simulink model "SIRModell"  (R2024b)
settings: Solver=VariableStepAuto  StartTime=0.0  StopTime=365  RelTol=1e-3
settings Model: Creator=castl  LastModifiedBy=castl

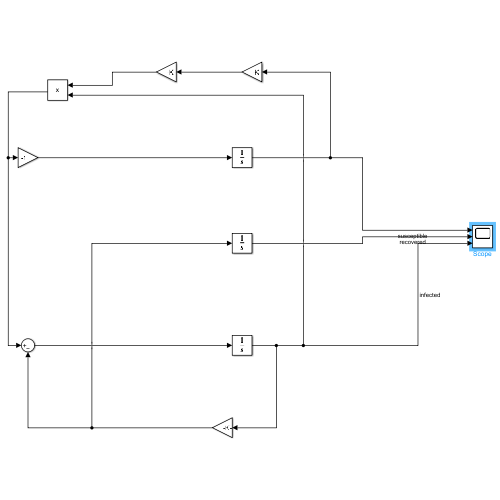
[thumbnail: Simulink's stored preview of the top-level diagram]
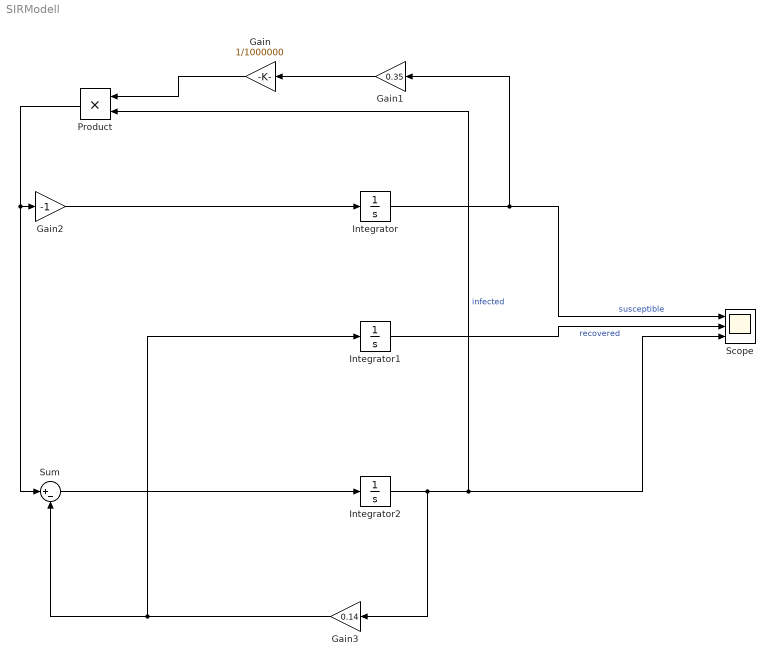
== system SIRModell ==
  Gain : Gain  Gain=1/1000000
  Gain1 : Gain  Gain=0.35
  Gain2 : Gain  Gain=-1
  Gain3 : Gain  Gain=0.14
  Integrator : Integrator  InitialCondition=999833
  Integrator1 : Integrator  InitialCondition=1
  Integrator2 : Integrator  InitialCondition=166
  Product : Product
  Scope : Scope  NumInputPorts=3
  Sum : Sum  Inputs=|+-
  wires:
  Gain2/1 -> Integrator/1
  Sum/1 -> Integrator2/1
  Gain3/1 -> Integrator1/1, Sum/2
  Integrator2/1 -> Gain3/1, Product/2, Scope/3  "infected"
  Integrator1/1 -> Scope/2  "recovered"
  Integrator/1 -> Gain1/1, Scope/1  "susceptible"
  Gain1/1 -> Gain/1
  Gain/1 -> Product/1
  Product/1 -> Sum/1, Gain2/1
